simulink library "DareLib"  (R2018b)
settings: Solver=VariableStepAuto  StartTime=0.0  StopTime=10.0  RelTol=1e-3
libraries: simulink x4, $bdroot x3
(part 2 of 2)

== stateflow chart DareLib/Dare/SeatHeight/SeatHeight ==
  state MotorSw
    en:
    MemSwCmd=0,SetPosi=0,SwCmd2=0,TmSwCmd=0,MotorRunTimeCnt=0,TMRunTimeCnt=0,MemToSWCnt=0,MemToMemCnt=0,TmtoTmCnt=0,SwDiffCnt=0,PreSWST=0,PreMEMST=0,PreTMST=0,SwDelay=10,MemSwFlg=0,TmMemSwCmd=0,TmFirstFlg=0,PreTmSetPosi=0;
    du:
    note: %当读取记忆档位位置成功后，并且按下记忆调用开关
    note: %TM模式下多次设置不同位置时，清TmFirstFlg标志
    note: %MemSwFlg是表示有记忆按键按下，避免按下时，没读记忆成功
    note: %记忆调用退出：电源模式处于 ON 档且档位处于非 P 档或 N 档
    note: %当电机停止后，并且电机控制关闭，才清除电机连续转动时间
    note: %当电机停止后，并且电机控制关闭，才清除电机连续转动时间
    note: %非记忆状态下，CRANK停止电机控制
    note: %正常结束时，清TmFirstFlg标志，允许下次调用
    note: %电机堵转 或 未获取上次的位置值或 电机连续转动时间超过20S， 停止电机，清记忆调用开关
    note: %电源模式处于CRANK，停止电机，但不清记忆调用开关
    note: %本地优先级大于记忆调用：执行本地开关，清记忆调用开关
    note: %记忆调用转本地：处于记忆调用，本地开关有效，停止电机100ms后，再执行本地开关
    note: %本地转本地：电机运动中，本地反向开关有效，停止电机100ms后，再执行反向电机
    note: %记忆调用转记忆调用：记忆运动中，记忆调用反向开关有效，停止电机100ms后，再执行反向电机
    MotorSw -> (junction 1868)
    (junction 1868) -> (junction 1848) [order 1] : [TmSwValid==0]
    (junction 1848) -> (junction 1660) [order 1] : [(SW==0)&&(MemSetValidFlg==0)&&((MemSw~=0)||(MemSwFlg==1))]
    (junction 1660) -> (junction 1873) : {SetPosi=posi;MemSwFlg=1;}
    (junction 1873) -> (junction 1861) [order 1] : [MemReadPosiFlg==1]
    (junction 1861) -> (junction 1835) [order 1] : [SetPosi > RealPosi]
    (junction 1868) -> (junction 1917) [order 2]
    (junction 1848) -> (junction 1645) [order 2]
    (junction 1873) -> (junction 1822) [order 2]
    (junction 1861) -> (junction 1663) [order 2] : {MemSwCmd=2;}
    (junction 1835) -> (junction 1688) : {MemSwCmd=1;}
    (junction 1917) -> (junction 1918) [order 1] : [PreTmSetPosi~=posi]
    (junction 1917) -> (junction 1922) [order 2]
    (junction 1918) -> (junction 1920) : {TmFirstFlg=0;}
    (junction 1822) -> (junction 1645)
    (junction 1663) -> (junction 1822) : {MemSwFlg=0;}
    (junction 1688) -> (junction 1663)
    (junction 1645) -> (junction 1667) : {TmMemSwCmd=0;
        | TMRunTimeCnt=0;
        | TmFirstFlg=0;}
    (junction 1920) -> (junction 1922)
    (junction 1922) -> (junction 1655)
    (junction 1667) -> (junction 1708) [order 1] : [MemSwCmd==1]
    (junction 1708) -> (junction 1901) : {SwCmd2=1;}
    (junction 1901) -> (junction 1860) [order 1] : [(SetPosi<=RealPosi)||(((TCU_GEAR~=1)&&(TCU_GEAR~=3))&&(POWER_MODE_BCM==2))]
    (junction 1655) -> (junction 1915) [order 1] : [TmFirstFlg==0]
    (junction 1915) -> (junction 1720) : {SetPosi=posi;
        | TMCmdFg=0;
        | TmFirstFlg=1;
        | PreTmSetPosi=SetPosi;}
    (junction 1720) -> (junction 1634) [order 1] : [SetPosi > RealPosi]
    (junction 1667) -> (junction 1758) [order 2]
    (junction 1901) -> (junction 1703) [order 2]
    (junction 1860) -> (junction 1780) : {
        | SwCmd2=0;
        | MemSwCmd=0;
        | }
    (junction 1655) -> (junction 1637) [order 2]
    (junction 1720) -> (junction 1724) [order 2] : {TmMemSwCmd=2;}
    (junction 1634) -> (junction 1808) : {TmMemSwCmd=1;}
    (junction 1758) -> (junction 1854) [order 1] : [MemSwCmd==2]
    (junction 1854) -> (junction 1856) : {SwCmd2=2;}
    (junction 1856) -> (junction 1760) [order 1] : [(SetPosi>=RealPosi)||(((TCU_GEAR~=1)&&(TCU_GEAR~=3))&&(POWER_MODE_BCM==2))]
    (junction 1758) -> (junction 1838) [order 2]
    (junction 1856) -> (junction 1815) [order 2]
    (junction 1760) -> (junction 1745) : {
        | SwCmd2=0;
        | MemSwCmd=0;
        | }
    (junction 1724) -> (junction 1637)
    (junction 1808) -> (junction 1724)
    (junction 1637) -> (junction 1752)
    (junction 1838) -> (junction 1644) [order 1] : [MemSwCmd==0]
    (junction 1838) -> (junction 1829) [order 2]
    (junction 1644) -> (junction 1772) : {SwCmd2=0;}
    (junction 1752) -> (junction 1643) [order 1] : [TmMemSwCmd==1]
    (junction 1643) -> (junction 1788) : {TmSwCmd=1;}
    (junction 1788) -> (junction 1698) [order 1] : [SetPosi<=RealPosi]
    (junction 1752) -> (junction 1894) [order 2]
    (junction 1788) -> (junction 1775) [order 2]
    (junction 1698) -> (junction 1694) : {
        | TmSwCmd=0;
        | TmMemSwCmd=0;
        | }
    (junction 1894) -> (junction 1803) [order 1] : [TmMemSwCmd==2]
    (junction 1803) -> (junction 1881) : {TmSwCmd=2;}
    (junction 1881) -> (junction 1719) [order 1] : [SetPosi>=RealPosi]
    (junction 1894) -> (junction 1696) [order 2]
    (junction 1881) -> (junction 1805) [order 2]
    (junction 1719) -> (junction 1807) : {
        | TmSwCmd=0;
        | TmMemSwCmd=0;
        | }
    (junction 1815) -> (junction 1772)
    (junction 1745) -> (junction 1815)
    (junction 1780) -> (junction 1703)
    (junction 1772) -> (junction 1829)
    (junction 1703) -> (junction 1745)
    (junction 1829) -> (junction 1813)
    (junction 1813) -> (junction 1784) [order 1] : [MemStopFg == 1]
    (junction 1813) -> (junction 1686) [order 2]
    (junction 1784) -> (junction 1863) : {SwCmd2=0;
        | MemSwCmd=0;}
    (junction 1696) -> (junction 1814) [order 1] : [TmMemSwCmd==0]
    (junction 1696) -> (junction 1678) [order 2]
    (junction 1814) -> (junction 1770) : {TmSwCmd=0;}
    (junction 1863) -> (junction 1686)
    (junction 1686) -> (junction 1728) : {SwCmd =SwCmd2; }
    (junction 1805) -> (junction 1770)
    (junction 1807) -> (junction 1805)
    (junction 1694) -> (junction 1775)
    (junction 1770) -> (junction 1678)
    (junction 1775) -> (junction 1807)
    (junction 1728) -> (junction 1707) [order 1] : [CurrST==1]
    (junction 1707) -> (junction 1727) : {MotorRunTimeCnt = MotorRunTimeCnt + 1;}
    (junction 1727) -> (junction 1726) [order 1] : [MotorRunTimeCnt >= MotorRunTimeOut]
    (junction 1678) -> (junction 1676) : {SwCmd =TmSwCmd; }
    (junction 1728) -> (junction 1668) [order 2]
    (junction 1727) -> (junction 1675) [order 2]
    (junction 1726) -> (junction 1712) : {MotorRunTimeCnt=MotorRunTimeOut;}
    (junction 1668) -> (junction 1832) [order 1] : [(CurrST==0)&&(SW==0)&&(SwCmd2==0)]
    (junction 1668) -> (junction 1766) [order 2]
    (junction 1832) -> (junction 1654) : {MotorRunTimeCnt=0;}
    (junction 1676) -> (junction 1812) [order 1] : [CurrST==1]
    (junction 1812) -> (junction 1795) : {TMRunTimeCnt = TMRunTimeCnt + 1;}
    (junction 1795) -> (junction 1632) [order 1] : [TMRunTimeCnt >= MotorRunTimeOut]
    (junction 1676) -> (junction 1767) [order 2]
    (junction 1795) -> (junction 1638) [order 2]
    (junction 1632) -> (junction 1779) : {TMRunTimeCnt=MotorRunTimeOut;}
    (junction 1654) -> (junction 1766)
    (junction 1675) -> (junction 1654)
    (junction 1712) -> (junction 1675)
    (junction 1766) -> (junction 1933)
    (junction 1767) -> (junction 1646) [order 1] : [(CurrST==0)&&(SW==0)&&(TmSwCmd==0)]
    (junction 1767) -> (junction 1888) [order 2]
    (junction 1646) -> (junction 1879) : {TMRunTimeCnt=0;}
    (junction 1879) -> (junction 1888)
    (junction 1638) -> (junction 1879)
    (junction 1779) -> (junction 1638)
    (junction 1888) -> (junction 1959)
    (junction 1933) -> (junction 1934) [order 1] : [(FaultST == 1)&&(SwCmd==1)]
    (junction 1933) -> (junction 1941) [order 2]
    (junction 1934) -> (junction 1936)
    (junction 1959) -> (junction 1970) [order 1] : [(FaultST == 1)&&(SwCmd==1)]
    (junction 1941) -> (junction 1943) [order 1] : [(FaultST == 2)&&(SwCmd==2)]
    (junction 1959) -> (junction 1962) [order 2]
    (junction 1970) -> (junction 1963)
    (junction 1941) -> (junction 1948) [order 2]
    (junction 1943) -> (junction 1945)
    (junction 1962) -> (junction 1979) [order 1] : [(FaultST == 2)&&(SwCmd==2)]
    (junction 1948) -> (junction 1950) [order 1] : [FaultST == 3]
    (junction 1962) -> (junction 1968) [order 2]
    (junction 1979) -> (junction 1964)
    (junction 1948) -> (junction 1956) [order 2]
    (junction 1950) -> (junction 1952)
    (junction 1968) -> (junction 1981) [order 1] : [FaultST == 3]
    (junction 1968) -> (junction 1973) [order 2]
    (junction 1981) -> (junction 1976)
    (junction 1952) -> (junction 1956) : {SwCmd=0;
        | MemSwCmd=0;
        | MemSwFlg=0;}
    (junction 1945) -> (junction 1952)
    (junction 1936) -> (junction 1945)
    (junction 1956) -> (junction 1743)
    (junction 1976) -> (junction 1973) : {SwCmd=0;
        | TmMemSwCmd=0;
        | MemSwFlg=0;}
    (junction 1964) -> (junction 1976)
    (junction 1963) -> (junction 1964)
    (junction 1973) -> (junction 1818)
    (junction 1743) -> (junction 1693) [order 1] : [(MemGetRTPosiFlg==0)||(MotorRunTimeCnt >= MotorRunTimeOut)]
    (junction 1743) -> (junction 1777) [order 2]
    (junction 1693) -> (junction 1850) : {MemSwCmd=0;
        | MemSwFlg=0;}
    (junction 1777) -> (junction 1665) [order 1] : [(POWER_MODE_BCM == 3)&&(SwCmd2==0)]
    (junction 1818) -> (junction 1636) [order 1] : [(MemGetRTPosiFlg==0)||(TMRunTimeCnt >= MotorRunTimeOut)]
    (junction 1777) -> (junction 1741) [order 2]
    (junction 1665) -> (junction 1889)
    (junction 1818) -> (junction 1700) [order 2]
    (junction 1636) -> (junction 1689) : {TmMemSwCmd=0;
        | MemSwFlg=0;
        | SwCmd=0;
        | TmtoTmCnt=0;}
    (junction 1741) -> (junction 1876) [order 1] : [SW~=0]
    (junction 1876) -> (junction 1884) [order 1] : [SwCmd2~=0]
    (junction 1884) -> (junction 1810) : {MemToSWCnt = MemToSWCnt + 1;}
    (junction 1810) -> (junction 1647) [order 1] : [MemToSWCnt>SwDelay]
    (junction 1700) -> (junction 1759) [order 1] : [TmSwCmd~=0]
    (junction 1759) -> (junction 1823) : [(PreTMST~=0)&&(PreTMST~=TmSwCmd)]
    (junction 1741) -> (junction 1677) [order 2]
    (junction 1876) -> (junction 1913) [order 2]
    (junction 1810) -> (junction 1744) [order 2] : {SwCmd=0;}
    (junction 1647) -> (junction 1722) : {MemToSWCnt=SwDelay;
        | SwCmd=SW;
        | MemSwCmd=0;
        | MemSwFlg=0;}
    (junction 1700) -> (junction 1842) [order 2] : {TmtoTmCnt=0;}
    (junction 1823) -> (junction 1846) : {TmtoTmCnt = TmtoTmCnt + 1;}
    (junction 1640) -> (junction 1796) : [(PreMEMST~=0)&&(PreMEMST~=SW)]
    (junction 1796) -> (junction 1702) : {MemToMemCnt = MemToMemCnt + 1;}
    (junction 1702) -> (junction 1789) [order 1] : [MemToMemCnt>SwDelay]
    (junction 1913) -> (junction 1875) [order 1] : [(PreSWST~=0)&&(PreSWST~=SW)]
    (junction 1875) -> (junction 1792) : {SwDiffCnt = SwDiffCnt + 1;}
    (junction 1792) -> (junction 1893) [order 1] : [SwDiffCnt>SwDelay]
    (junction 1677) -> (junction 1640) [order 1] : [SwCmd2~=0]
    (junction 1702) -> (junction 1809) [order 2] : {SwCmd=0;}
    (junction 1789) -> (junction 1669) : {
        | MemToMemCnt=SwDelay;
        | SwCmd=SwCmd2;
        | }
    (junction 1913) -> (junction 1737) [order 2] : {SwCmd=SW;
        | MemSwCmd=0;
        | MemSwFlg=0;}
    (junction 1792) -> (junction 1905) [order 2] : {SwCmd=0;}
    (junction 1893) -> (junction 1692) : {SwDiffCnt=SwDelay;
        | SwCmd=SW;
        | PreSWST=SwCmd;}
    (junction 1677) -> (junction 1738) [order 2] : {SwDiffCnt=0;
        | MemToSWCnt=0;
        | MemToMemCnt=0;}
    (junction 1846) -> (junction 1906) [order 1] : [TmtoTmCnt>SwDelay]
    (junction 1846) -> (junction 1887) [order 2] : {SwCmd=0;}
    (junction 1906) -> (junction 1769) : {
        | TmtoTmCnt=SwDelay;
        | SwCmd=TmSwCmd;
        | }
    (junction 1887) -> (junction 1842)
    (junction 1769) -> (junction 1887)
    (junction 1689) -> (junction 1769)
    (junction 1842) -> (junction 1886) : {PreTMST=TmSwCmd;}
    (junction 1886) -> (junction 1731) [order 1] : [(TmMemSwCmd==0)&&(SwCmd==0)]
    (junction 1886) -> (junction 1717) [order 2]
    (junction 1731) -> (junction 1729) : {TMCmdFg=1;
        | TmFirstFlg=0;}
    (junction 1809) -> (junction 1738)
    (junction 1669) -> (junction 1809)
    (junction 1737) -> (junction 1669)
    (junction 1905) -> (junction 1737)
    (junction 1692) -> (junction 1905)
    (junction 1744) -> (junction 1692)
    (junction 1722) -> (junction 1744)
    (junction 1889) -> (junction 1722) : {SwCmd=0;}
    (junction 1850) -> (junction 1889)
    (junction 1738) -> (junction 1713) : {PreSWST=SW;
        | PreMEMST=SwCmd2;}
    (junction 1729) -> (junction 1717)
    (junction 1717) -> (junction 1685)
    (junction 1685) -> (junction 1713)
    (junction 1713) -> (junction 1706)
  data: SW input; CurrST input; MemSw input; RealPosi input; SetPosi local uint16; MemSwCmd local uint8; SwCmd output; SwCmd2 local uint8; POWER_MODE_BCM input; posi input; MemGetRTPosiFlg input; MemReadPosiFlg input; MotorRunTimeCnt local uint16; SwDiffCnt local uint16; MemToSWCnt local uint16; PreSWST local uint8; SwDelay local uint16; MemSwFlg local boolean; FaultST input; TCU_GEAR input; MemSetValidFlg input; MemToMemCnt local uint16; PreMEMST local uint8; TmSwValid input; TmSwCmd local uint16; TmtoTmCnt local uint16; PreTMST local uint8; TMRunTimeCnt local uint16; TmMemSwCmd local uint16; MemStopFg input; MotorRunTimeOut input; TMCmdFg output; PreTmSetPosi local uint16; TmFirstFlg local boolean
